simulink model "RoverSimulation"  (R2024b)
settings: Solver=VariableStepAuto  StartTime=0.0  StopTime=10.0  RelTol=1e-3
settings Model: Creator=turnwald  LastModifiedBy=turnwald

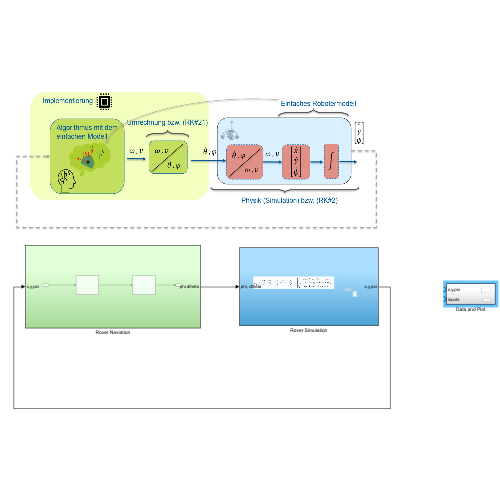
[thumbnail: Simulink's stored preview of the top-level diagram]
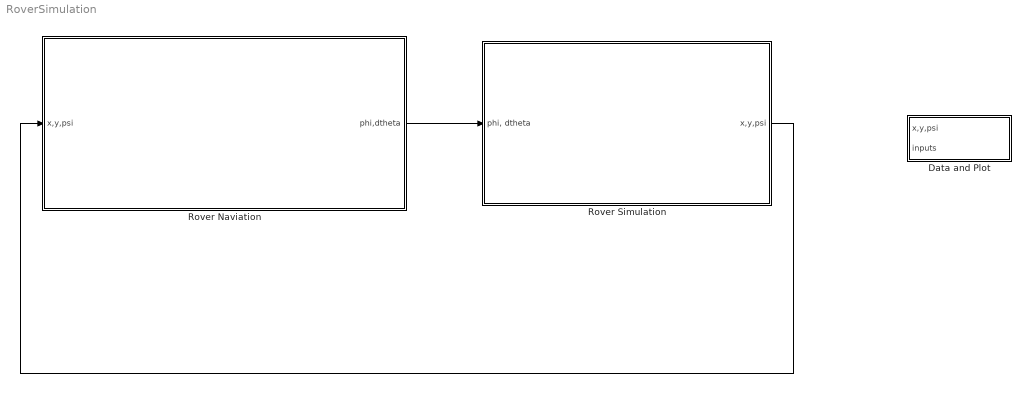
== system RoverSimulation ==
  Data and Plot : Subsystem
  Rover Naviation : Subsystem
  Rover Simulation : Subsystem
  wires:
  Rover Simulation/1(x,y,psi) -> Rover Naviation/1(x,y,psi)
  Rover Naviation/1(phi,dtheta) -> Rover Simulation/1("phi, dtheta")

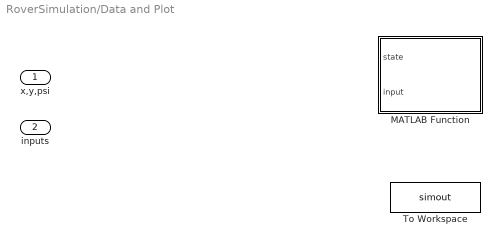
== system RoverSimulation/Data and Plot ==
  x,y,psi : Inport
  inputs : Inport  Port=2
  MATLAB Function : MATLAB Function  TreatAsAtomicUnit=on
  To Workspace : ToWorkspace  VariableName=simout  SaveFormat=Timeseries  SampleTime=-1

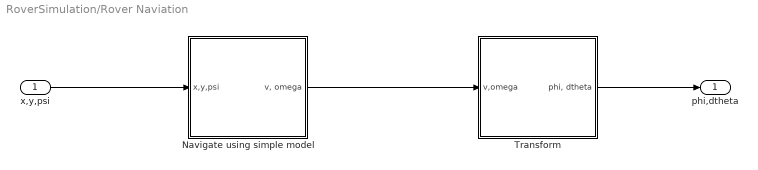
== system RoverSimulation/Rover Naviation ==
  x,y,psi : Inport
  Navigate using simple model : Subsystem
  Transform : Subsystem
  phi,dtheta : Outport
  wires:
  x,y,psi/1 -> Navigate using simple model/1(x,y,psi)
  Transform/1("phi, dtheta") -> phi,dtheta/1
  Navigate using simple model/1("v, omega") -> Transform/1(v,omega)

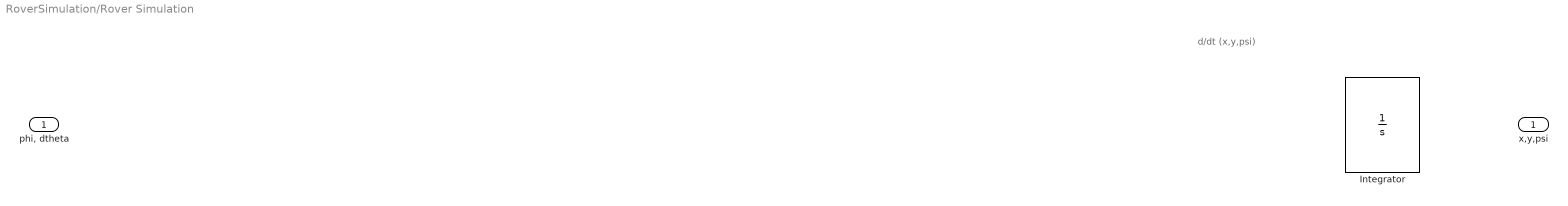
== system RoverSimulation/Rover Simulation ==
  note: d/dt (x,y,psi)
  "phi, dtheta" : Inport
  Integrator : Integrator
  x,y,psi : Outport

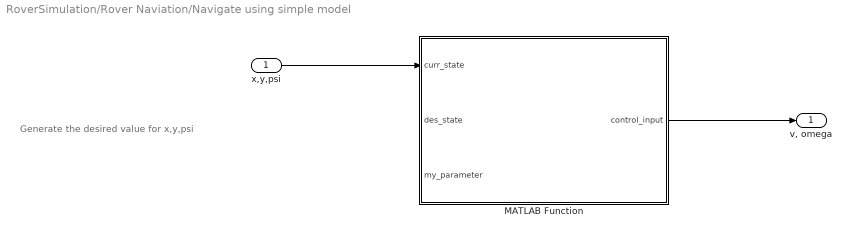
== system RoverSimulation/Rover Naviation/Navigate using simple model ==
  note: Generate the desired value for x,y,psi
  x,y,psi : Inport
  MATLAB Function : MATLAB Function  TreatAsAtomicUnit=on
  "v, omega" : Outport
  wires:
  x,y,psi/1 -> MATLAB Function/1(curr_state)
  ? -> MATLAB Function/2(des_state)
  MATLAB Function/1(control_input) -> "v, omega"/1

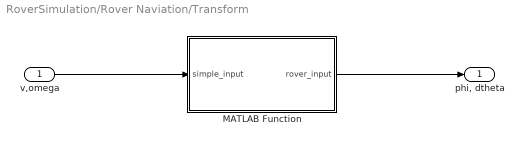
== system RoverSimulation/Rover Naviation/Transform ==
  v,omega : Inport
  MATLAB Function : MATLAB Function  TreatAsAtomicUnit=on
  "phi, dtheta" : Outport
  wires:
  v,omega/1 -> MATLAB Function/1(simple_input)
  MATLAB Function/1(rover_input) -> "phi, dtheta"/1

== matlab function RoverSimulation/Rover Naviation/Navigate using simple model/MATLAB Function ==
  data: curr_state input; control_input output; des_state input; my_parameter input
function control_input = navigate_to_desired_point(curr_state, des_state, my_parameter)

control_input = 0;

== matlab function RoverSimulation/Data and Plot/MATLAB Function ==
  data: state input; input input
function plot(state,input)

coder.extrinsic('plot_a_rover')

plot_a_rover(state,input);
pause(0.1);

== matlab function RoverSimulation/Rover Naviation/Transform/MATLAB Function ==
  data: simple_input input; rover_input output
function rover_input = fcn(simple_input)

rover_input = 0;
